simulink model "ControllerValidationHarness"  (R2025b)
settings: Solver=ode4  StartTime=0.0  StopTime=protocol.t(end)  FixedStep=Ts  RelTol=1e-3
undefined symbols (not defined in the file): A_ctrl, A_obs_k, A_obs_l, B_ctrl, B_obs_k, B_obs_l, C_ctrl, C_obs_k, C_obs_l, D_ctrl, D_obs_k, D_obs_l, feedback_selector_id, k1_smc, k2_smc, K_eq_smc, phi_smc, S_smc, SB_smc, smc_int_ic, theta_uff_gain, theta_xss_gain, ud_neg, ud_pos, V_sat_hw
settings Model: Creator=U448565  LastModifiedBy=U448565

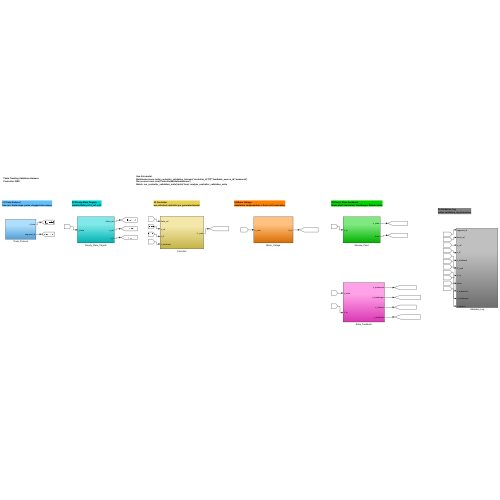
[thumbnail: Simulink's stored preview of the top-level diagram]
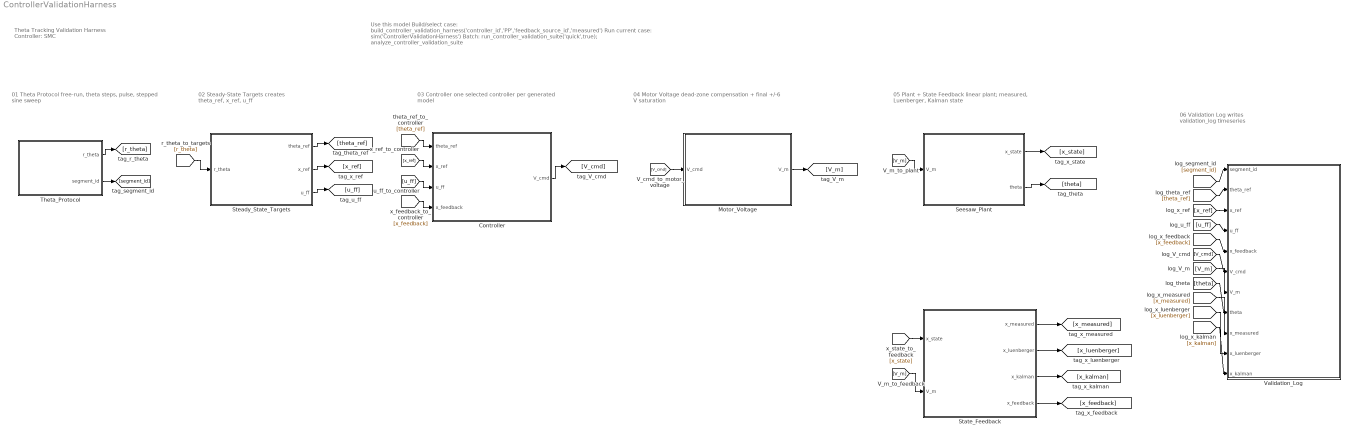
== system ControllerValidationHarness ==
  note: Theta Tracking Validation Harness
      | Controller: SMC
  note: Use this model
      | Build/select case: build_controller_validation_harness('controller_id','PP','feedback_source_id','measured')
      | Run current case: sim('ControllerValidationHarness')
      | Batch: run_controller_validation_suite('quick',true); analyze_controller_validation_suite
  note: 01 Theta Protocol
      | free-run, theta steps, pulse, stepped sine sweep
  note: 02 Steady-State Targets
      | creates theta_ref, x_ref, u_ff
  note: 03 Controller
      | one selected controller per generated model
  note: 04 Motor Voltage
      | dead-zone compensation + final +/-6 V saturation
  note: 05 Plant + State Feedback
      | linear plant; measured, Luenberger, Kalman state
  note: 06 Validation Log
      | writes validation_log timeseries
  Controller : Subsystem
  Motor_Voltage : Subsystem
  Seesaw_Plant : Subsystem
  State_Feedback : Subsystem
  Steady_State_Targets : Subsystem
  Theta_Protocol : Subsystem
  Validation_Log : Subsystem
  wires:
  Theta_Protocol/1(r_theta) -> [r_theta]
  Theta_Protocol/2(segment_id) -> [segment_id]
  Steady_State_Targets/1(theta_ref) -> [theta_ref]
  Steady_State_Targets/2(x_ref) -> [x_ref]
  Steady_State_Targets/3(u_ff) -> [u_ff]
  Controller/1(V_cmd) -> [V_cmd]
  Motor_Voltage/1(V_m) -> [V_m]
  Seesaw_Plant/1(x_state) -> [x_state]
  Seesaw_Plant/2(theta) -> [theta]
  State_Feedback/1(x_measured) -> [x_measured]
  State_Feedback/2(x_luenberger) -> [x_luenberger]
  State_Feedback/3(x_kalman) -> [x_kalman]
  State_Feedback/4(x_feedback) -> [x_feedback]
  [r_theta] -> Steady_State_Targets/1(r_theta)
  [theta_ref] -> Controller/1(theta_ref)
  [x_ref] -> Controller/2(x_ref)
  [u_ff] -> Controller/3(u_ff)
  [x_feedback] -> Controller/4(x_feedback)
  [V_cmd] -> Motor_Voltage/1(V_cmd)
  [V_m] -> Seesaw_Plant/1(V_m)
  [x_state] -> State_Feedback/1(x_state)
  [V_m] -> State_Feedback/2(V_m)
  [segment_id] -> Validation_Log/1(segment_id)
  [theta_ref] -> Validation_Log/2(theta_ref)
  [x_ref] -> Validation_Log/3(x_ref)
  [u_ff] -> Validation_Log/4(u_ff)
  [x_feedback] -> Validation_Log/5(x_feedback)
  [V_cmd] -> Validation_Log/6(V_cmd)
  [V_m] -> Validation_Log/7(V_m)
  [theta] -> Validation_Log/8(theta)
  [x_measured] -> Validation_Log/9(x_measured)
  [x_luenberger] -> Validation_Log/10(x_luenberger)
  [x_kalman] -> Validation_Log/11(x_kalman)

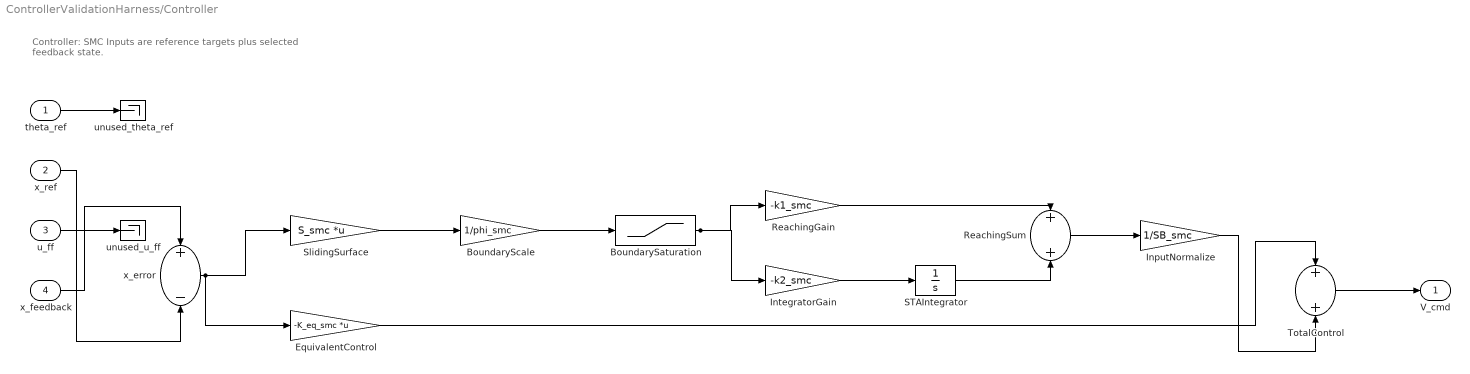
== system ControllerValidationHarness/Controller ==
  note: Controller: SMC
      | Inputs are reference targets plus selected feedback state.
  theta_ref : Inport
  x_ref : Inport  Port=2
  u_ff : Inport  Port=3
  x_feedback : Inport  Port=4
  BoundarySaturation : Saturate  UpperLimit=1  LowerLimit=-1
  BoundaryScale : Gain  Gain=1/phi_smc
  EquivalentControl : Gain  Gain=-K_eq_smc  Multiplication=Matrix(K*u)
  InputNormalize : Gain  Gain=1/SB_smc
  IntegratorGain : Gain  Gain=-k2_smc
  ReachingGain : Gain  Gain=-k1_smc
  ReachingSum : Sum
  STAIntegrator : Integrator  InitialCondition=smc_int_ic
  SlidingSurface : Gain  Gain=S_smc  Multiplication=Matrix(K*u)
  TotalControl : Sum
  unused_theta_ref : Terminator
  unused_u_ff : Terminator
  x_error : Sum  Inputs=+-
  V_cmd : Outport
  wires:
  theta_ref/1 -> unused_theta_ref/1
  u_ff/1 -> unused_u_ff/1
  x_feedback/1 -> x_error/1
  x_ref/1 -> x_error/2
  x_error/1 -> SlidingSurface/1, EquivalentControl/1
  SlidingSurface/1 -> BoundaryScale/1
  BoundaryScale/1 -> BoundarySaturation/1
  BoundarySaturation/1 -> ReachingGain/1, IntegratorGain/1
  IntegratorGain/1 -> STAIntegrator/1
  ReachingGain/1 -> ReachingSum/1
  STAIntegrator/1 -> ReachingSum/2
  ReachingSum/1 -> InputNormalize/1
  EquivalentControl/1 -> TotalControl/1
  InputNormalize/1 -> TotalControl/2
  TotalControl/1 -> V_cmd/1

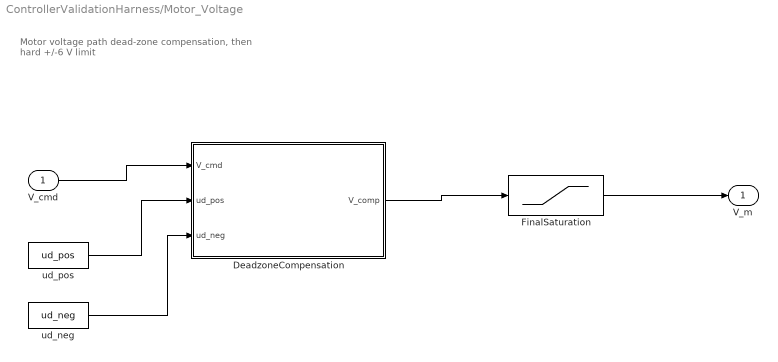
== system ControllerValidationHarness/Motor_Voltage ==
  note: Motor voltage path
      | dead-zone compensation, then hard +/-6 V limit
  V_cmd : Inport
  DeadzoneCompensation : MATLAB Function  TreatAsAtomicUnit=on
  FinalSaturation : Saturate  UpperLimit=V_sat_hw  LowerLimit=-V_sat_hw
  ud_neg : Constant  Value=ud_neg
  ud_pos : Constant  Value=ud_pos
  V_m : Outport
  wires:
  V_cmd/1 -> DeadzoneCompensation/1(V_cmd)
  ud_pos/1 -> DeadzoneCompensation/2(ud_pos)
  ud_neg/1 -> DeadzoneCompensation/3(ud_neg)
  DeadzoneCompensation/1(V_comp) -> FinalSaturation/1
  FinalSaturation/1 -> V_m/1

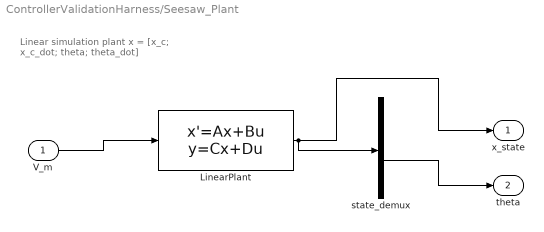
== system ControllerValidationHarness/Seesaw_Plant ==
  note: Linear simulation plant
      | x = [x_c; x_c_dot; theta; theta_dot]
  V_m : Inport
  LinearPlant : StateSpace  A=A_ctrl  B=B_ctrl  C=C_ctrl  D=D_ctrl  InitialCondition=[0;0;0;0]
  state_demux : Demux
  x_state : Outport
  theta : Outport  Port=2
  wires:
  V_m/1 -> LinearPlant/1
  LinearPlant/1 -> x_state/1, state_demux/1
  state_demux/3 -> theta/1

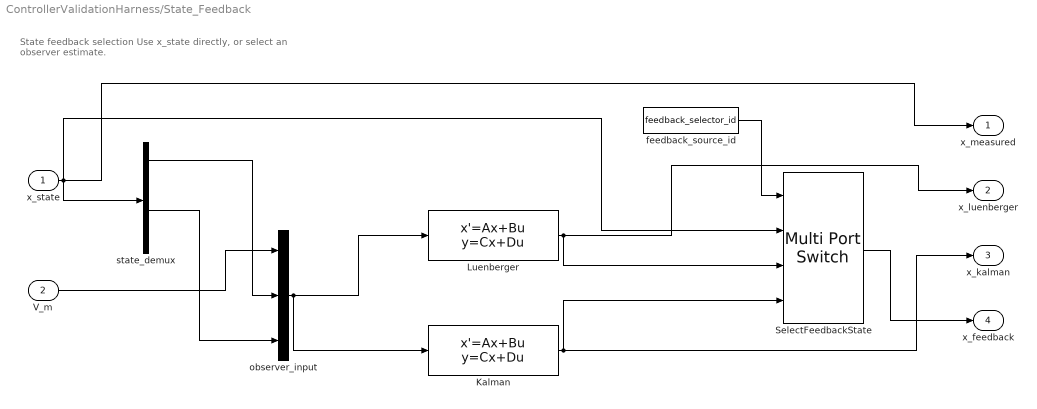
== system ControllerValidationHarness/State_Feedback ==
  note: State feedback selection
      | Use x_state directly, or select an observer estimate.
  x_state : Inport
  V_m : Inport  Port=2
  Kalman : StateSpace  A=A_obs_k  B=B_obs_k  C=C_obs_k  D=D_obs_k  InitialCondition=[0;0;0;0]
  Luenberger : StateSpace  A=A_obs_l  B=B_obs_l  C=C_obs_l  D=D_obs_l  InitialCondition=[0;0;0;0]
  SelectFeedbackState : MultiPortSwitch  SaturateOnIntegerOverflow=off  InputSameDT=off
  feedback_source_id : Constant  Value=feedback_selector_id
  observer_input : Mux  Inputs=3
  state_demux : Demux
  x_measured : Outport
  x_luenberger : Outport  Port=2
  x_kalman : Outport  Port=3
  x_feedback : Outport  Port=4
  wires:
  x_state/1 -> x_measured/1, state_demux/1, SelectFeedbackState/2
  V_m/1 -> observer_input/1
  state_demux/1 -> observer_input/2
  state_demux/3 -> observer_input/3
  observer_input/1 -> Luenberger/1, Kalman/1
  Luenberger/1 -> x_luenberger/1, SelectFeedbackState/3
  Kalman/1 -> x_kalman/1, SelectFeedbackState/4
  feedback_source_id/1 -> SelectFeedbackState/1
  SelectFeedbackState/1 -> x_feedback/1

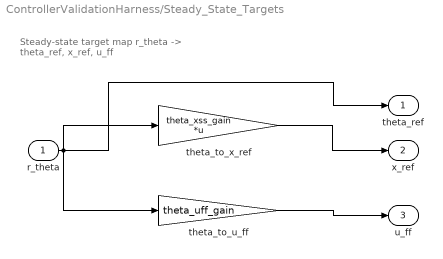
== system ControllerValidationHarness/Steady_State_Targets ==
  note: Steady-state target map
      | r_theta -> theta_ref, x_ref, u_ff
  r_theta : Inport
  theta_to_u_ff : Gain  Gain=theta_uff_gain
  theta_to_x_ref : Gain  Gain=theta_xss_gain  Multiplication=Matrix(K*u)
  theta_ref : Outport
  x_ref : Outport  Port=2
  u_ff : Outport  Port=3
  wires:
  r_theta/1 -> theta_ref/1, theta_to_x_ref/1, theta_to_u_ff/1
  theta_to_x_ref/1 -> x_ref/1
  theta_to_u_ff/1 -> u_ff/1

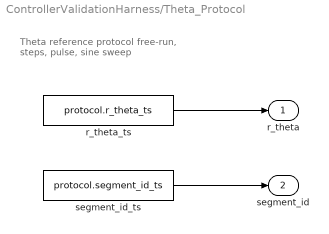
== system ControllerValidationHarness/Theta_Protocol ==
  note: Theta reference protocol
      | free-run, steps, pulse, sine sweep
  r_theta_ts : FromWorkspace  VariableName=protocol.r_theta_ts
  segment_id_ts : FromWorkspace  VariableName=protocol.segment_id_ts
  r_theta : Outport
  segment_id : Outport  Port=2
  wires:
  r_theta_ts/1 -> r_theta/1
  segment_id_ts/1 -> segment_id/1

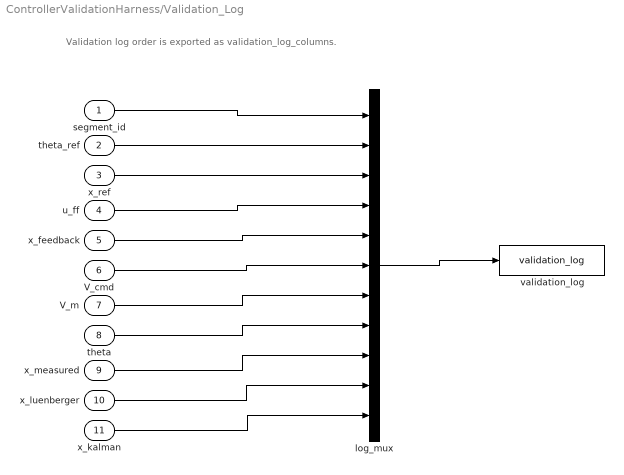
== system ControllerValidationHarness/Validation_Log ==
  note: Validation log order is exported as validation_log_columns.
  segment_id : Inport
  theta_ref : Inport  Port=2
  x_ref : Inport  Port=3
  u_ff : Inport  Port=4
  x_feedback : Inport  Port=5
  V_cmd : Inport  Port=6
  V_m : Inport  Port=7
  theta : Inport  Port=8
  x_measured : Inport  Port=9
  x_luenberger : Inport  Port=10
  x_kalman : Inport  Port=11
  log_mux : Mux  Inputs=11
  validation_log : ToWorkspace  VariableName=validation_log  SaveFormat=Timeseries  SampleTime=-1
  wires:
  segment_id/1 -> log_mux/1
  theta_ref/1 -> log_mux/2
  x_ref/1 -> log_mux/3
  u_ff/1 -> log_mux/4
  x_feedback/1 -> log_mux/5
  V_cmd/1 -> log_mux/6
  V_m/1 -> log_mux/7
  theta/1 -> log_mux/8
  x_measured/1 -> log_mux/9
  x_luenberger/1 -> log_mux/10
  x_kalman/1 -> log_mux/11
  log_mux/1 -> validation_log/1

== matlab function ControllerValidationHarness/Motor_Voltage/DeadzoneCompensation ==
  data: V_cmd input; V_comp output; ud_pos input; ud_neg input
function V_comp = fcn(V_cmd, ud_pos, ud_neg)
% Add just enough voltage to overcome measured motor dead-zone.
threshold = 0.1;
if V_cmd > threshold
    V_comp = V_cmd + ud_pos;
elseif V_cmd < -threshold
    V_comp = V_cmd - ud_neg;
else
    V_comp = 0;
end
